simulink model "RLC"  (R2016a)
settings: Solver=VariableStepAuto  StartTime=0.0  StopTime=10.0  RelTol=1e-3
settings Model: Creator=cinlab  LastModifiedBy=cinlab

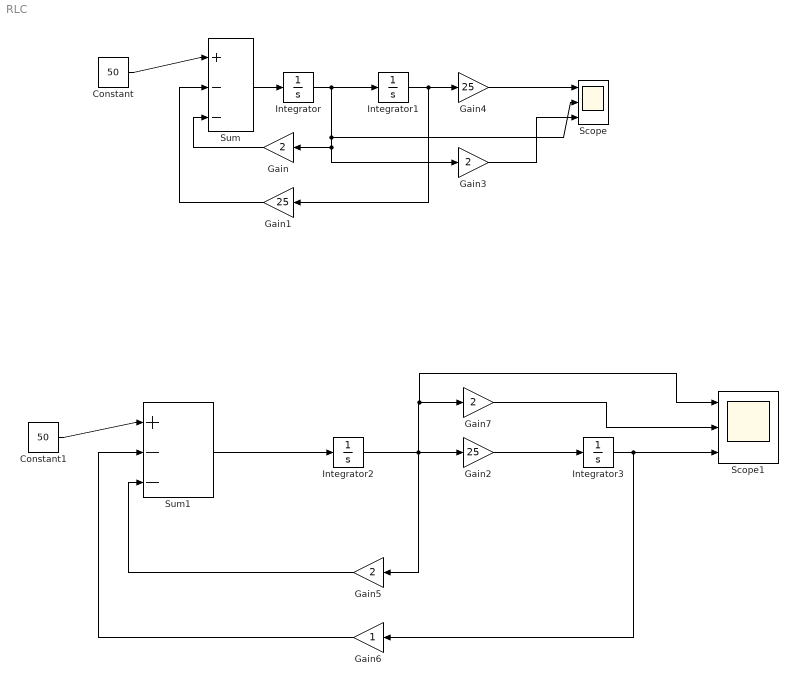
== system RLC ==
  Constant : Constant  Value=50
  Constant1 : Constant  Value=50
  Gain{,3,5,7} (4 alike) : Gain  Gain=2
  Gain1 : Gain  Gain=25
  Gain2 : Gain  Gain=25
  Gain4 : Gain  Gain=25
  Gain6 : Gain
  Integrator{,1..3} (4 alike) : Integrator
  Scope : Scope  NumInputPorts=3
  Scope1 : Scope  NumInputPorts=3
  Sum : Sum  Inputs=|+--
  Sum1 : Sum  Inputs=|+--
  wires:
  Sum/1 -> Integrator/1
  Integrator/1 -> Integrator1/1, Scope/2, Gain3/1, Gain/1
  Gain/1 -> Sum/3
  Gain1/1 -> Sum/2
  Constant/1 -> Sum/1
  Integrator1/1 -> Gain4/1, Gain1/1
  Gain4/1 -> Scope/1
  Gain3/1 -> Scope/3
  Sum1/1 -> Integrator2/1
  Integrator2/1 -> Scope1/1, Gain7/1, Gain5/1, Gain2/1
  Gain2/1 -> Integrator3/1
  Gain5/1 -> Sum1/3
  Gain6/1 -> Sum1/2
  Integrator3/1 -> Scope1/3, Gain6/1
  Constant1/1 -> Sum1/1
  Gain7/1 -> Scope1/2
